simulink model "pendbasic2"  (R2015b)
settings: Solver=ode5  StartTime=0.0  StopTime=100  FixedStep=h  RelTol=1e-3
values from neighbouring files (symbols this model uses):
  Fscomp_neg = 0.16    [pendinit.m]
  Fscomp_pos = 0.16    [pendinit.m]
  g = 9.81    [pendinit.m]
  h = 0.01    [pendinit.m]
  Lnopos = dlqr(Afd,Bfd,Q,R)    [pendinit.m]
  Lpos = dlqr(Afd,Bfd,Q,R)    [pendinit.m]
undefined symbols (not defined in the file): J, Jp, l, m, M, r, x0
settings Model: ExtModeTrigMode=oneshot  ExtModeArmWhenConnect=off  ExtModeAutoUpdateStatusClock=off  Creator=lincoln  LastModifiedBy=Jonathan
settings DataIOCC: LimitDataPoints=off  SaveFormat=Array  SignalLoggingSaveFormat=ModelDataLogs
settings OptimizationCC: BooleanDataType=off  ExpressionDepthLimit=2147483647  InitFltsAndDblsToZero=on
settings DebuggingCC: SaveWithParameterizedLinksMsg=none  UnderspecifiedInitializationDetection=Classic  MergeDetectMultiDrivingBlocksExec=none  SignalResolutionControl=TryResolveAllWithWarning  MultiTaskDSMMsg=warning  MultiTaskCondExecSysMsg=none  FcnCallInpInsideContextMsg=UseLocalSettings  StateNameClashWarn=warning
settings HardwareCC: ProdBitPerPointer=32  ProdLargestAtomicFloat=None  ProdIntDivRoundTo=Undefined  ProdEndianess=Unspecified  ProdWordSize=32  ProdHWDeviceType=32-bit Generic  TargetUnknown=on
settings GRTTargetCC: GeneratePreprocessorConditionals=Disable all  CombineOutputUpdateFcns=off  GRTInterface=on
settings ConfigComp: CovModelRefEnable=Off

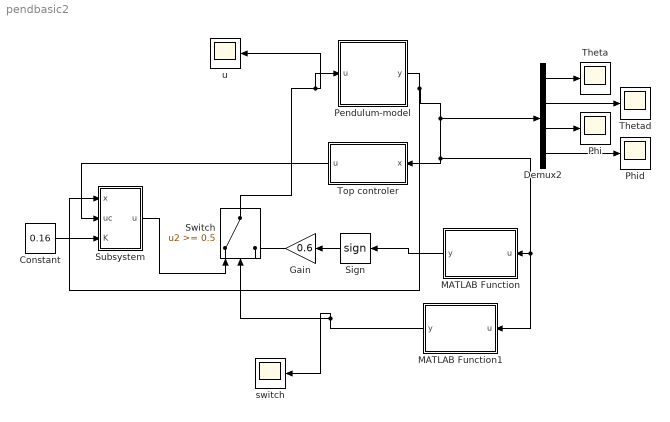
== system pendbasic2 ==
  Constant : Constant  Value=0.16
  Demux2 : Demux
  Gain : Gain  Gain=0.6
  MATLAB Function : MATLAB Function  TreatAsAtomicUnit=on
  MATLAB Function1 : MATLAB Function  TreatAsAtomicUnit=on
  Pendulum-model : Subsystem
      mask Display: disp('Model')
  Phi : Scope
  Phid : Scope
  Sign : Signum
  Subsystem : Subsystem
  Switch : Switch  Threshold=0.5
  Theta : Scope
  Thetad : Scope
  Top controler : Subsystem
  switch : Scope
  u : Scope
  wires:
  Demux2/2 -> Thetad/1
  Demux2/3 -> Phi/1
  Demux2/4 -> Phid/1
  Demux2/1 -> Theta/1
  Pendulum-model/1(y) -> Subsystem/1(x), Demux2/1, Top controler/1(x), MATLAB Function/1(u), MATLAB Function1/1(u)
  MATLAB Function/1(y) -> Sign/1
  Sign/1 -> Gain/1
  MATLAB Function1/1(y) -> switch/1, Switch/2
  Switch/1 -> u/1, Pendulum-model/1(u)
  Gain/1 -> Switch/3
  Top controler/1(u) -> Subsystem/2(uc)
  Subsystem/1(u) -> Switch/1
  Constant/1 -> Subsystem/3(K)

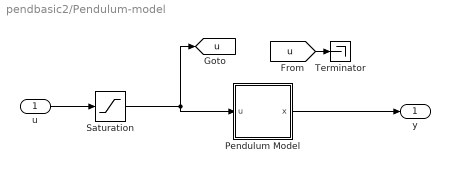
== system pendbasic2/Pendulum-model ==
  u : Inport
  Pendulum Model : Subsystem
  Saturation : Saturate  UpperLimit=2  LowerLimit=-2
  Terminator : Terminator
  y : Outport  InitialOutput=0
  tag scope: u=global
  wires:
  Saturation/1 -> Pendulum Model/1(u), [u]
  u/1 -> Saturation/1
  [u] -> Terminator/1
  Pendulum Model/1(x) -> y/1

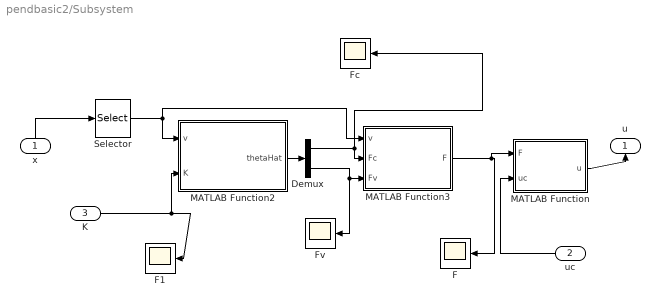
== system pendbasic2/Subsystem ==
  x : Inport
  uc : Inport  Port=2
  K : Inport  Port=3
  Demux : Demux  Outputs=2
  F : Scope
  F1 : Scope
  Fc : Scope
  Fv : Scope
  MATLAB Function : MATLAB Function  TreatAsAtomicUnit=on
  MATLAB Function2 : MATLAB Function  TreatAsAtomicUnit=on
  MATLAB Function3 : MATLAB Function  TreatAsAtomicUnit=on
  Selector : Selector  InputPortWidth=4  IndexOptions=Index vector (dialog)  Indices=4  OutputSizes=1
  u : Outport
  wires:
  x/1 -> Selector/1
  uc/1 -> MATLAB Function/2(uc)
  K/1 -> F1/1, MATLAB Function2/2(K)
  Selector/1 -> MATLAB Function3/1(v), MATLAB Function2/1(v)
  Demux/2 -> Fv/1, MATLAB Function3/3(Fv)
  MATLAB Function2/1(thetaHat) -> Demux/1
  Demux/1 -> Fc/1, MATLAB Function3/2(Fc)
  MATLAB Function3/1(F) -> MATLAB Function/1(F), F/1
  MATLAB Function/1(u) -> u/1

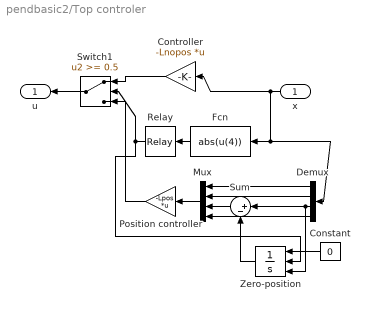
== system pendbasic2/Top controler ==
  x : Inport
  Constant : Constant  Value=0
  Controller : Gain  Gain=-Lnopos  Multiplication=Matrix(K*u)  SaturateOnIntegerOverflow=on  OutDataTypeStr=Inherit: Same as input  ParamDataTypeStr=Inherit: Same as input
  Demux : Demux
  Fcn : Fcn  Expr=abs(u(4))
  Mux : Mux
  Position controller : Gain  Gain=-Lpos  Multiplication=Matrix(K*u)  SaturateOnIntegerOverflow=on  OutDataTypeStr=Inherit: Same as input  ParamDataTypeStr=Inherit: Same as input
  Relay : Relay  OnSwitchValue=4  OffSwitchValue=3.9
  Sum : Sum  Inputs=|+-  SaturateOnIntegerOverflow=on  InputSameDT=on  OutDataTypeStr=Inherit: Same as first input
  Switch1 : Switch  Threshold=0.5  SaturateOnIntegerOverflow=on  InputSameDT=on
  Zero-position : Integrator  ExternalReset=falling  InitialConditionSource=external
  u : Outport
  wires:
  Switch1/1 -> u/1
  Sum/1 -> Mux/3
  Zero-position/1 -> Sum/2
  Fcn/1 -> Relay/1
  Constant/1 -> Zero-position/1
  Demux/3 -> Sum/1, Zero-position/3
  Demux/4 -> Mux/4
  Demux/2 -> Mux/2
  Demux/1 -> Mux/1
  Mux/1 -> Position controller/1
  Controller/1 -> Switch1/1
  Relay/1 -> Switch1/2, Zero-position/2
  Position controller/1 -> Switch1/3
  x/1 -> Controller/1, Demux/1, Fcn/1

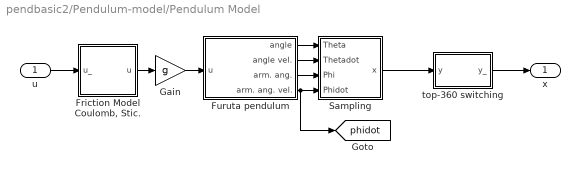
== system pendbasic2/Pendulum-model/Pendulum Model ==
  u : Inport
  "Friction Model Coulomb, Stic." : Subsystem
  Furuta pendulum : Subsystem  mask{l=l, M=M, Jp=Jp, r=r, J=J, m_w=m, g=g, x_0=x0}
      mask prompts: l "Pendulum Length"; M "Mass of Pendulum"; r "Length of Arm"; m_w "Mass of weight"
  Gain : Gain  Gain=g  SaturateOnIntegerOverflow=on  OutDataTypeStr=Inherit: Same as input  ParamDataTypeStr=Inherit: Same as input
  Sampling : Subsystem
  top-360 switching : Subsystem
  x : Outport  InitialOutput=0
  tag scope: phidot=global
  wires:
  Gain/1 -> Furuta pendulum/1(u)
  "Friction Model Coulomb, Stic."/1(u) -> Gain/1
  u/1 -> "Friction Model Coulomb, Stic."/1(u_)
  Furuta pendulum/4(arm. ang. vel.) -> [phidot], Sampling/4(Phidot)
  Furuta pendulum/2(angle vel.) -> Sampling/2(Thetadot)
  Furuta pendulum/3(arm. ang.) -> Sampling/3(Phi)
  Furuta pendulum/1(angle) -> Sampling/1(Theta)
  Sampling/1(x) -> top-360 switching/1(y)
  top-360 switching/1(y_) -> x/1

== system pendbasic2/Pendulum-model/Pendulum Model/Friction Model Coulomb, Stic. ==
  u_ : Inport
  Friction model : Subsystem
  u : Outport  InitialOutput=0
  wires:
  u_/1 -> Friction model/1(u)
  [phidot] -> Friction model/2(phidot)
  Friction model/1(u_) -> u/1

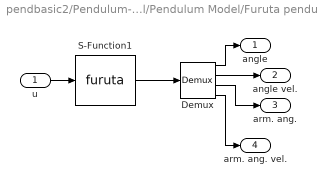
== system pendbasic2/Pendulum-model/Pendulum Model/Furuta pendulum ==
  u : Inport
  Demux : Demux
  S-Function1 : S-Function  FunctionName=furuta  Parameters=l, M, Jp, r, J, m_w, g, x_0  SFunctionDeploymentMode=off  EnableBusSupport=off
  angle : Outport  InitialOutput=0
  angle vel. : Outport  Port=2  InitialOutput=0
  arm. ang. : Outport  Port=3  InitialOutput=0
  arm. ang. vel. : Outport  Port=4  InitialOutput=0
  wires:
  S-Function1/1 -> Demux/1
  Demux/1 -> angle/1
  Demux/2 -> angle vel./1
  u/1 -> S-Function1/1
  Demux/3 -> arm. ang./1
  Demux/4 -> arm. ang. vel./1

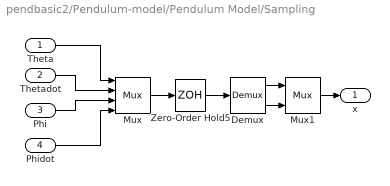
== system pendbasic2/Pendulum-model/Pendulum Model/Sampling ==
  Theta : Inport
  Thetadot : Inport  Port=2
  Phi : Inport  Port=3
  Phidot : Inport  Port=4
  Demux : Demux  Outputs=[3 1]
  Mux : Mux
  Mux1 : Mux  Inputs=2
  Zero-Order Hold5 : ZeroOrderHold  SampleTime=h
  x : Outport  InitialOutput=0
  wires:
  Demux/1 -> Mux1/1
  Mux1/1 -> x/1
  Zero-Order Hold5/1 -> Demux/1
  Mux/1 -> Zero-Order Hold5/1
  Phidot/1 -> Mux/4
  Phi/1 -> Mux/3
  Thetadot/1 -> Mux/2
  Theta/1 -> Mux/1
  Demux/2 -> Mux1/2

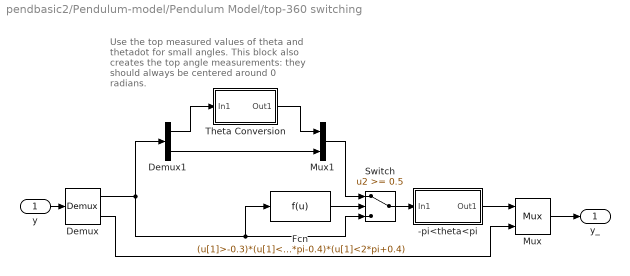
== system pendbasic2/Pendulum-model/Pendulum Model/top-360 switching ==
  note: Use the top measured values of
      | theta and thetadot for small angles.
      | This block also creates the top angle
      | measurements: they should always be
      | centered around 0 radians.
  y : Inport
  -pi<theta<pi : Subsystem
  Demux : Demux  Outputs=[2 2]
  Demux1 : Demux  Outputs=2
  Fcn : Fcn  Expr=(u[1]>-0.3)*(u[1]<0.4)+(u[1]>2*pi-0.4)*(u[1]<2*pi+0.4)
  Mux : Mux  Inputs=2
  Mux1 : Mux  Inputs=2
  Switch : Switch  Threshold=0.5  SaturateOnIntegerOverflow=on  InputSameDT=on
  Theta Conversion : Subsystem
  y_ : Outport
  wires:
  -pi<theta<pi/1(Out1) -> Mux/1
  Switch/1 -> -pi<theta<pi/1(In1)
  Theta Conversion/1(Out1) -> Mux1/1
  Fcn/1 -> Switch/2
  Mux/1 -> y_/1
  y/1 -> Demux/1
  Demux/2 -> Mux/2
  Demux/1 -> Demux1/1, Switch/3, Fcn/1
  Demux1/1 -> Theta Conversion/1(In1)
  Demux1/2 -> Mux1/2
  Mux1/1 -> Switch/1

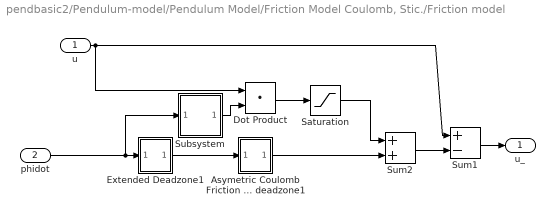
== system pendbasic2/Pendulum-model/Pendulum Model/Friction Model Coulomb, Stic./Friction model ==
  u : Inport
  phidot : Inport  Port=2
  Asymetric Coulomb Friction with deadzone1 : Subsystem  mask{Fc_neg=Fscomp_neg, Fc_pos=Fscomp_pos, dv=0.04}
      mask prompts: Fc_neg "Coulomb Friction (Negative)"; Fc_pos "Coulomb Friction (Positive)"; dv "Deadzone width (Onesided)"
      mask Display:
      | plot([-1 0 0], [0 0 1], [0 0 1],[-1 0 0]);
      | plot([0.5 0.5 1],[0 0.5 0.5],[-0.5 -0.5 -1],[0 -0.5 -0.5]);
  Dot Product : DotProduct  InputSameDT=on  OutDataTypeStr=Inherit: Inherit via internal rule
  Extended Deadzone1 : Subsystem  mask{vg=1, dv=0.04}
      mask prompts: vg "Gain"; dv "Deadzone width (Onesided)"
      mask init:
      | v_gain=vg;
      | d_v=dv;
      mask Display:
      | plot([-1 0 0], [0 0 1], [0 0 1],[-1 0 0]);
      | plot([0.5 0.5 1],[0 0.5 1],[-0.5 -0.5 -1],[0 -0.5 -1]);
  Saturation : Saturate  UpperLimit=Fscomp_pos  LowerLimit=-Fscomp_neg
  Subsystem : Subsystem  mask{dw=0.04}
      mask prompts: dw "Width (Onesided)"
      mask init:
      | d_w=dw;
      mask Display:
      | plot([-1 0 0], [0 0 1], [0 0 1],[-0.3 0 0]);
      | plot([-0.5 -0.5 0.5 0.5],[0 0.7 0.7 0])
  Sum1 : Sum  Inputs=+-  SaturateOnIntegerOverflow=on  InputSameDT=on  OutDataTypeStr=Inherit: Same as first input
  Sum2 : Sum  SaturateOnIntegerOverflow=on  InputSameDT=on  OutDataTypeStr=Inherit: Same as first input
  u_ : Outport  InitialOutput=0
  wires:
  Saturation/1 -> Sum2/1
  phidot/1 -> Extended Deadzone1/1(In1), Subsystem/1(In1)
  Sum1/1 -> u_/1
  Extended Deadzone1/1(Out1) -> Asymetric Coulomb Friction with deadzone1/1(In1)
  Subsystem/1(Out1) -> Dot Product/2
  Dot Product/1 -> Saturation/1
  u/1 -> Dot Product/1, Sum1/1
  Sum2/1 -> Sum1/2
  Asymetric Coulomb Friction with deadzone1/1(Out1) -> Sum2/2

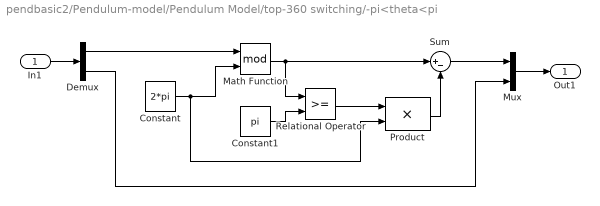
== system pendbasic2/Pendulum-model/Pendulum Model/top-360 switching/-pi<theta<pi ==
  In1 : Inport
  Constant : Constant  Value=2*pi
  Constant1 : Constant  Value=pi
  Demux : Demux  Outputs=2
  Math Function : Math  Operator=mod  SaturateOnIntegerOverflow=on
  Mux : Mux  Inputs=2
  Product : Product  SaturateOnIntegerOverflow=on  RndMeth=Zero  InputSameDT=on  OutDataTypeStr=Inherit: Same as first input
  Relational Operator : RelationalOperator  InputSameDT=on
  Sum : Sum  Inputs=|+-  SaturateOnIntegerOverflow=on  InputSameDT=on  OutDataTypeStr=Inherit: Same as first input
  Out1 : Outport
  wires:
  Demux/2 -> Mux/2
  Mux/1 -> Out1/1
  Sum/1 -> Mux/1
  Demux/1 -> Math Function/1
  In1/1 -> Demux/1
  Product/1 -> Sum/2
  Relational Operator/1 -> Product/1
  Constant1/1 -> Relational Operator/2
  Math Function/1 -> Relational Operator/1, Sum/1
  Constant/1 -> Product/2, Math Function/2

== system pendbasic2/Pendulum-model/Pendulum Model/top-360 switching/Theta Conversion ==
  In1 : Inport
  Fcn1 : Fcn  Expr=(u[1]-u[2])*2*pi-pi
  Fcn2 : Fcn  Expr=u/(2*pi)-1/2
  Mux : Mux  Inputs=2
  Rounding Function : Rounding
  Out1 : Outport  InitialOutput=0
  wires:
  In1/1 -> Fcn2/1
  Fcn1/1 -> Out1/1
  Mux/1 -> Fcn1/1
  Fcn2/1 -> Mux/1, Rounding Function/1
  Rounding Function/1 -> Mux/2

== system pendbasic2/Pendulum-model/Pendulum Model/Friction Model Coulomb, Stic./Friction model/Asymetric Coulomb Friction with deadzone1 ==
  In1 : Inport
  Dead Zone : DeadZone  LowerValue=-dv  UpperValue=dv  SaturateOnIntegerOverflow=on
  Fcn : Fcn  Expr=(u<0)*u*Fc_neg+(u>0)*u*Fc_pos
  Sign : Signum
  Out1 : Outport  InitialOutput=0
  wires:
  Fcn/1 -> Out1/1
  Sign/1 -> Fcn/1
  Dead Zone/1 -> Sign/1
  In1/1 -> Dead Zone/1

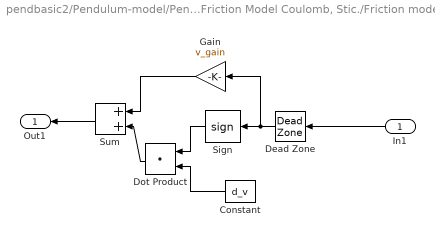
== system pendbasic2/Pendulum-model/Pendulum Model/Friction Model Coulomb, Stic./Friction model/Extended Deadzone1 ==
  In1 : Inport
  Constant : Constant  Value=d_v
  Dead Zone : DeadZone  LowerValue=-d_v  UpperValue=d_v  SaturateOnIntegerOverflow=on
  Dot Product : DotProduct  InputSameDT=on  OutDataTypeStr=Inherit: Inherit via internal rule
  Gain : Gain  Gain=v_gain  SaturateOnIntegerOverflow=on  OutDataTypeStr=Inherit: Same as input  ParamDataTypeStr=Inherit: Same as input
  Sign : Signum
  Sum : Sum  SaturateOnIntegerOverflow=on  InputSameDT=on  OutDataTypeStr=Inherit: Same as first input
  Out1 : Outport  InitialOutput=0
  wires:
  Gain/1 -> Sum/1
  In1/1 -> Dead Zone/1
  Sign/1 -> Dot Product/1
  Dead Zone/1 -> Gain/1, Sign/1
  Constant/1 -> Dot Product/2
  Dot Product/1 -> Sum/2
  Sum/1 -> Out1/1

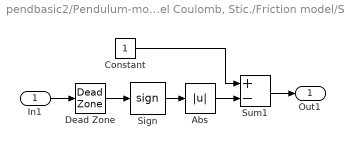
== system pendbasic2/Pendulum-model/Pendulum Model/Friction Model Coulomb, Stic./Friction model/Subsystem ==
  In1 : Inport
  Abs : Abs  SaturateOnIntegerOverflow=on
  Constant : Constant
  Dead Zone : DeadZone  LowerValue=-d_w  UpperValue=d_w  SaturateOnIntegerOverflow=on
  Sign : Signum
  Sum1 : Sum  Inputs=+-  SaturateOnIntegerOverflow=on  InputSameDT=on  OutDataTypeStr=Inherit: Same as first input
  Out1 : Outport  InitialOutput=0
  wires:
  Dead Zone/1 -> Sign/1
  In1/1 -> Dead Zone/1
  Constant/1 -> Sum1/1
  Sum1/1 -> Out1/1
  Sign/1 -> Abs/1
  Abs/1 -> Sum1/2

== matlab function pendbasic2/MATLAB Function1 ==
  data: u input; y output
function y = fcn(u)
%#codegen
ar=sqrt(0.62^2+9.4^2);
ar=ar*0.2;
br=sqrt(0.19^2+2.5^2);
br=br*0.2;
alfar=atan(9.4/0.62);
X = u(1);
Y = u(2);

term1 = X*cos(alfar)+Y*sin(alfar);
term2 = -X*sin(alfar) + Y*cos(alfar);
y = (term1^2/ar^2 + term2^2/br^2) < 1.5;
%y = abs(u(1)) + abs(u(2)) < 0.8;

== matlab function pendbasic2/MATLAB Function ==
  data: u input; y output
function y = fcn(u)
%#codegen
omega0 =  2*pi*0.9002;
y = cos(u(1))*u(2)*(cos(u(1))-1+u(2).^2/2/omega0^2);

== matlab function pendbasic2/Subsystem/MATLAB Function2 ==
  data: v input; K input; thetaHat output
function thetaHat = rls(v, K)
persistent P theta phi
if isempty(P)
    P =  eye(2)*1000;
    theta = [0; 0];
    phi = [0; 0];
end
P = (P-(P*phi*phi'*P)/(1+phi'*P*phi));
e = K-phi'*theta;
theta = theta + P*phi*e;
thetaHat = theta;
phi = [sign(v); v];
return

== matlab function pendbasic2/Subsystem/MATLAB Function3 ==
  data: v input; Fc input; F output; Fv input
function F = fcn(v, Fc, Fv)
F = Fc*sign(v)+Fv*v;
end

== matlab function pendbasic2/Subsystem/MATLAB Function ==
  data: u output; F input; uc input
function u = fcn(F,uc)
u=sign(uc) * abs(F) + uc;
end
